simulink model "MyPiero_EvitaObstaculos"  (R2022b)
settings: Solver=FixedStepDiscrete  StartTime=0.0  StopTime=10.0  RelTol=1e-3  EnableMultiTasking=on
model workspace (MAT data in the model file):
  d = 0.18
settings Model: ExtModeTrigDuration=2  Creator=Usuario  LastModifiedBy=Usuario
settings OptimizationCC: ReuseModelBlockBuffer=on  EnhancedBackFolding=on  PassReuseOutputArgsAs=Individual arguments  ZeroExternalMemoryAtStartup=off  ZeroInternalMemoryAtStartup=off  MaxStackSize=64  OptimizeBlockOrder=speed  DifferentSizesBufferReuse=on  EfficientTunableParamExpr=on
settings DebuggingCC: ParameterTunabilityLossMsg=error
settings HardwareCC: ProdBitPerInt=16  ProdBitPerPointer=16  ProdBitPerSizeT=16  ProdBitPerPtrDiffT=16  ProdLargestAtomicFloat=None  ProdWordSize=8  ProdHWDeviceType=Atmel->AVR  UseEmbeddedCoderFeatures=off  UseSimulinkCoderFeatures=off
settings SFSimCC: MATLABDynamicMemAlloc=off
settings RTWCC: Description=Embedded Coder  SystemTargetFile=ert.tlc  HardwareBoard=Arduino Mega 2560  TLCOptions=-aInlineSetEventsForThisBaseRateFcn=TLC_FALSE -aSuppressMultiTaskScheduler=TLC_FALSE -aRateBasedStepFcn=1  TemplateMakefile=ert_default_tmf  Toolchain=Arduino AVR  BuildConfiguration=Faster Runs  GPUComputeCapability=5.0
settings CodeAppCC: ForceParamTrailComments=on  IgnoreCustomStorageClasses=off  OperatorAnnotations=on  SimulinkDataObjDesc=on  SFDataObjDesc=on  MangleLength=10  InsertBlockDesc=on
settings ERTTargetCC: SupportContinuousTime=on  SupportNonInlinedSFcns=on  SupportVariableSizeSignals=on  ExtModeTransport=3  ExtModeStaticAlloc=on  ExtModeAutomaticAllocSize=off  ExtModeStaticAllocSize=2048  ExtModeMexFile=ext_xcp  ExtModeIntrfLevel=Level2 - Open

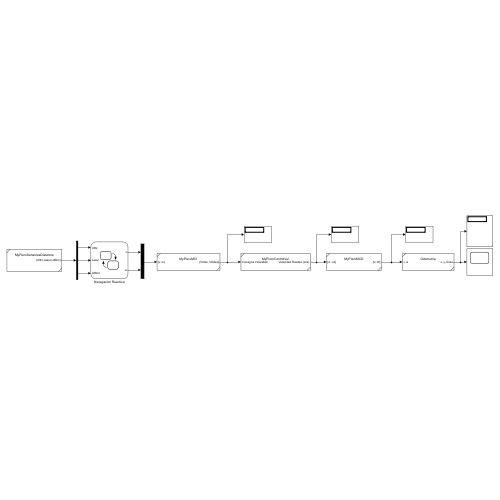
[thumbnail: Simulink's stored preview of the top-level diagram]
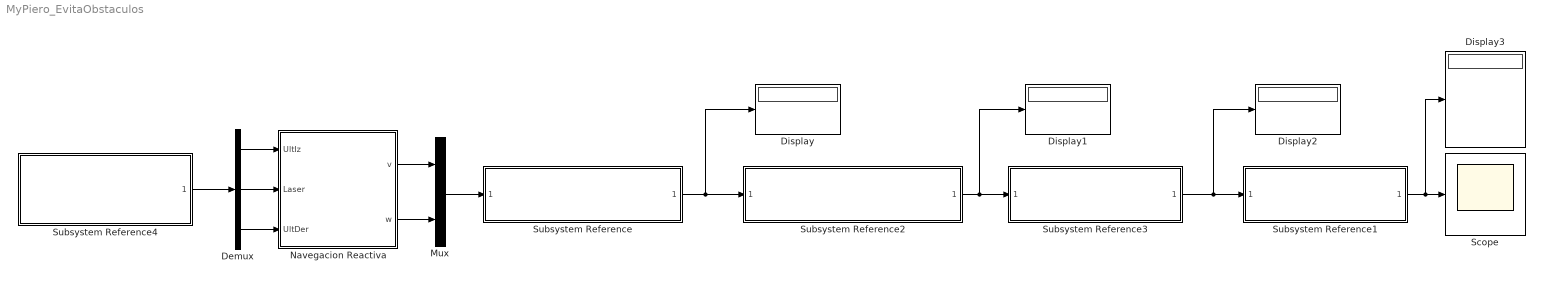
== system MyPiero_EvitaObstaculos ==
  Demux : Demux  Outputs=3
  Display{,1..3} (4 alike) : Display
  Mux : Mux  Inputs=2
  Navegacion Reactiva : Stateflow chart  TreatAsAtomicUnit=on
  Scope : Scope
  Subsystem Reference : Subsystem  ReferencedSubsystem=MyPieroMCI
  Subsystem Reference1 : Subsystem  ReferencedSubsystem=Odometria
  Subsystem Reference2 : Subsystem  ReferencedSubsystem=MyPieroControlVel
  Subsystem Reference3 : Subsystem  ReferencedSubsystem=MyPieroMCD
  Subsystem Reference4 : Subsystem  ReferencedSubsystem=MyPieroSensoresDistancia
  wires:
  Subsystem Reference3/1 -> Display2/1, Subsystem Reference1/1
  Subsystem Reference2/1 -> Display1/1, Subsystem Reference3/1
  Subsystem Reference/1 -> Display/1, Subsystem Reference2/1
  Subsystem Reference1/1 -> Display3/1, Scope/1
  Navegacion Reactiva/1(v) -> Mux/1
  Navegacion Reactiva/2(w) -> Mux/2
  Mux/1 -> Subsystem Reference/1
  Subsystem Reference4/1 -> Demux/1
  Demux/1 -> Navegacion Reactiva/1(UltIz)
  Demux/2 -> Navegacion Reactiva/2(Laser)
  Demux/3 -> Navegacion Reactiva/3(UltDer)

== stateflow chart MyPiero_EvitaObstaculos/Navegacion Reactiva ==
  state TightWay
    % Con esto intentare que
    % pase por un camino
    % estrecho hasta donde
    % pueda
    entry:
    v = 0.5;
    w = 0;
  state FullRotation
    % Si detecta algo
    % en todos los sentidos
    entry:
    v = 0;
    w = -pi + 0.1;
  state Default
    entry:
    v = 0.3;
    w = 0;
  state LeftSonar_Far
    % Si solo detecta el
    % Obstaculo con el
    % ultrasonidos izquierdo
    % lejos
    entry:
    v = 0.2;
    w = -pi/8;
  state LeftSonar_Close
    % Si solo detecta el
    % Obstaculo con el
    % ultrasonidos izquierdo
    % cerca
    entry:
    v = 0;
    w = -pi/4;
  state MidLaser
    entry:
    v = 0;
    w = 0;
    % Calculo el signo para
    % la rotacion aleatoria
    if round(rand) == 0
    sign = -1;
    else
    sign = 1;
    end
  state RightSonar_Close
    % Si solo detecta el
    % Obstaculo con el
    % ultrasonidos derecho
    % cerca
    entry:
    v = 0;
    w = pi/4;
  state RightSonar_Far
    % Si solo detecta el
    % Obstaculo con el
    % ultrasonidos izquierdo
    % lejos
    entry:
    v = 0.2;
    w = pi/8;
  state RandomRotation
    % Si solo detecta el
    % Obstaculo con el
    % Laser
    entry:
    v =  0;
    w = sign*pi/4;
  TightWay -> TightWay [order 2] : [(UltIz > 12) && (UltDer >12)]
  Default -> TightWay [order 2] : [(UltIz < 25) && (Laser >= 20) && (UltDer < 25)]
  TightWay -> FullRotation [order 3] : [(UltIz <= 12) && (UltDer <= 12)]
  TightWay -> Default [order 1] : after(0.1,sec)
  FullRotation -> FullRotation [order 1] : [Laser < 25]
  Default -> FullRotation [order 1] : [(UltIz < 25) && (Laser < 20) && (UltDer < 25)]
  FullRotation -> Default [order 2] : after(0.1, sec)
  (default) -> Default
  Default -> RightSonar_Far [order 5] : [(UltDer < 30) && (UltDer >= 20)]
  Default -> LeftSonar_Far [order 4] : [(UltIz < 30) && (UltIz >= 20)]
  RightSonar_Far -> Default [order 1] : [(UltDer >= 30) || (UltDer < 20)]
  LeftSonar_Far -> Default [order 1] : [(UltIz >= 30) || (UltIz < 20)]
  RightSonar_Close -> Default [order 1] : [UltDer >= 20]
  LeftSonar_Close -> Default [order 1] : [UltIz >= 20 ]
  Default -> RightSonar_Close [order 7] : [UltDer < 20]
  Default -> LeftSonar_Close [order 6] : [UltIz < 20]
  Default -> MidLaser [order 3] : [Laser < 20]
  MidLaser -> Default [order 1] : [Laser > 25]
  LeftSonar_Far -> LeftSonar_Far [order 2] : [(UltIz < 30) && (UltIz >= 20)]
  RightSonar_Far -> RightSonar_Far [order 2] : [(UltDer < 30) && (UltDer >= 20)]
  LeftSonar_Close -> LeftSonar_Close [order 2] : [UltIz < 20]
  RightSonar_Close -> RightSonar_Close [order 2] : [UltDer < 20]
  MidLaser -> RandomRotation [order 2] : after(0.1,sec)
  RandomRotation -> MidLaser [order 1] : after(0.2,sec)
  RandomRotation -> RandomRotation [order 2] : [Laser <= 25]
  data: UltIz input; Laser input; UltDer input; v output; w output; sign local
